simulink model "fuzzy_Control_sim"  (R2023a)
settings: Solver=VariableStepAuto  StartTime=0.0  StopTime=20  RelTol=1e-3
values from neighbouring files (symbols this model uses):
  c = 2050    [PID_Controller.m]    (also in set_Fun.m)
  ks = 60000    [PID_Controller.m]    (also in set_Fun.m)
  kt = 362000    [PID_Controller.m]    (also in set_Fun.m)
  ms = 1173    [PID_Controller.m]    (also in set_Fun.m)
  mu = 152.1    [PID_Controller.m]    (also in set_Fun.m)
undefined symbols (not defined in the file or in its folder): c0
libraries: fuzblock x2
settings Model: Creator=Administrator  LastModifiedBy=Administrator

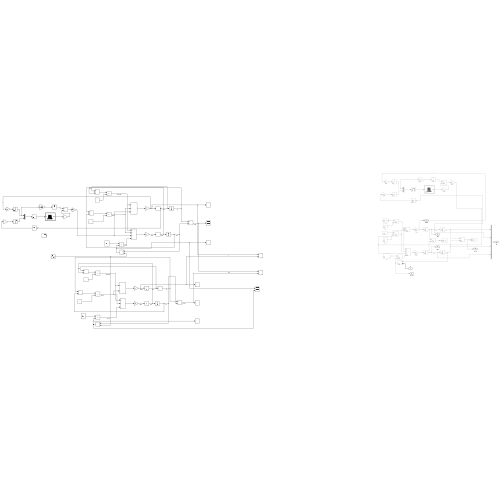
[thumbnail: Simulink's stored preview of the top-level diagram]
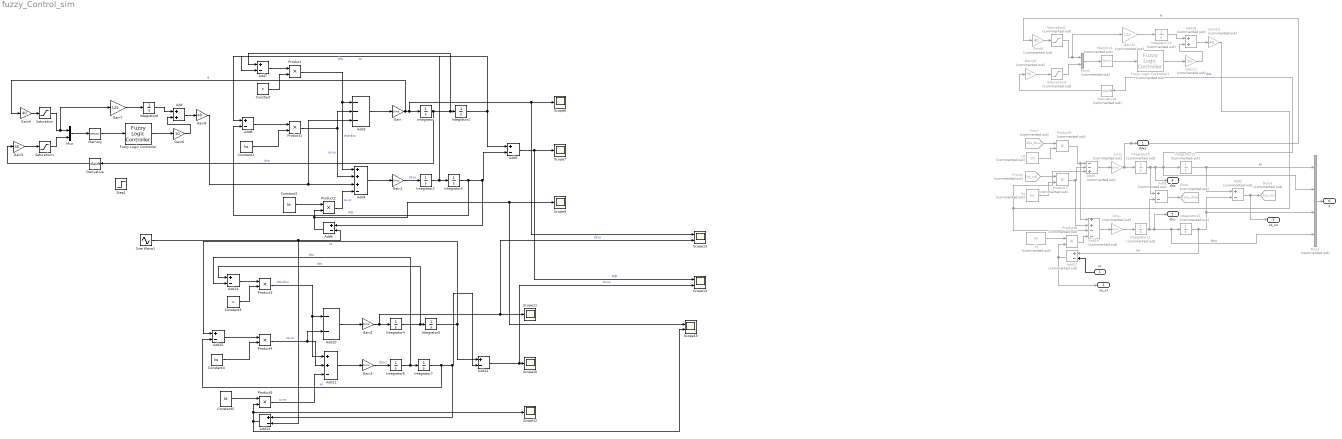
== system fuzzy_Control_sim ==
  xr : Inport
  1/ms : Gain  Commented=on  Gain=1/ms
  1/mu : Gain  Commented=on  Gain=1/mu
  Add : Sum
  Add1 : Sum  Commented=on  Inputs=+-
  Add10 : Sum  Inputs=--
  Add11 : Sum  Inputs=++-
  Add{5..8,12..15} (8 alike) : Sum  Inputs=+-
  Add16 : Sum  Commented=on  Inputs=++--
  Add17 : Sum  Commented=on  Inputs=+-
  Add18 : Sum  Commented=on
  Add2 : Sum  Commented=on  Inputs=+-
  Add3 : Sum  Inputs=---
  Add4 : Sum  Inputs=+++-
  Add9 : Sum  Commented=on  Inputs=--+
  Constant : Constant  Value=c
  Constant1 : Constant  Value=ks
  Constant2 : Constant  Value=kt
  Constant3 : Constant  Value=c
  Constant4 : Constant  Value=ks
  Constant5 : Constant  Value=kt
  Derivative : Derivative
  Derivative1 : Derivative  Commented=on
  From : From  Commented=on  GotoTag=dxs_dxu
  From2 : From  Commented=on  GotoTag=xs_xu
  Fuzzy Logic Controller : fuzblock/Fuzzy Logic  Controller  FIS='fuzzy_Model_1.fis'  OutputSampleNumber=101  DataType=double  FuzzifiedInputs=off  RuleFiringStrengths=off  RuleOutputs=off  AggregatedOutputs=off  SimulateUsing=Interpreted execution  OutOfRangeInputValueMessage=warning  NoRuleFiredMessage=warning  EmptyOutputFuzzySetMessage=warning
  Fuzzy Logic Controller1 : fuzblock/Fuzzy Logic  Controller  Commented=on  FIS='fuzzy_Model_1.fis'  OutputSampleNumber=101  DataType=double  FuzzifiedInputs=off  RuleFiringStrengths=off  RuleOutputs=off  AggregatedOutputs=off  SimulateUsing=Interpreted execution  OutOfRangeInputValueMessage=warning  NoRuleFiredMessage=warning  EmptyOutputFuzzySetMessage=warning
  Gain : Gain  Gain=1/ms
  Gain1 : Gain  Gain=1/mu
  Gain10 : Gain  Commented=on  Gain=30
  Gain11 : Gain  Commented=on  Gain=10
  Gain12 : Gain  Commented=on  Gain=125
  Gain13 : Gain  Commented=on  Gain=40
  Gain2 : Gain  Gain=1/ms
  Gain3 : Gain  Gain=1/mu
  Gain4 : Gain  Gain=40
  Gain5 : Gain  Gain=30
  Gain6 : Gain  Gain=10
  Gain7 : Gain  Gain=125
  Gain8 : Gain  Gain=40
  Gain9 : Gain  Commented=on  Gain=40
  Goto : Goto  Commented=on  GotoTag=dxs_dxu
  Goto1 : Goto  Commented=on  GotoTag=xs_xu
  Integrator{,1..8} (9 alike) : Integrator
  Integrator{9..13} (5 alike) : Integrator  Commented=on
  Memory : Memory  InitialCondition=1
  Memory1 : Memory  Commented=on  InitialCondition=1
  Mux : Mux  Inputs=2
  Mux1 : Mux  Commented=on
  Mux2 : Mux  Commented=on  Inputs=2
  Product{,1..5} (6 alike) : Product
  Product6 : Product  Commented=on
  Product7 : Product  Commented=on
  Product8 : Product  Commented=on
  Saturation : Saturate  UpperLimit=3  LowerLimit=-3
  Saturation1 : Saturate  UpperLimit=3  LowerLimit=-3
  Saturation2 : Saturate  Commented=on  UpperLimit=3  LowerLimit=-3
  Saturation3 : Saturate  Commented=on  UpperLimit=3  LowerLimit=-3
  Scope{7..12} (6 alike) : Scope
  Scope13 : Scope  NumInputPorts=2
  Scope14 : Scope  NumInputPorts=2
  Scope15 : Scope  NumInputPorts=2
  Sine Wave1 : Sin  Amplitude=0.05  Frequency=2*pi  SampleTime=0
  Step1 : Step  Time=0.1  SampleTime=0
  c0 : Constant  Commented=on  Value=c0
  ks : Constant  Commented=on  Value=ks
  kt : Constant  Commented=on  Value=kt
  ddxs : Outport
  xu_xr : Outport  Port=2
  xs_xu : Outport  Port=3
  dxs : Outport  Port=4
  dxu : Outport  Port=5
  X : Outport  Port=6
  wires:
  Add3/1 -> Gain/1
  Add4/1 -> Gain1/1
  Gain/1 -> Integrator/1, Scope13/1, Scope8/1, Gain4/1  "e"
  Gain1/1 -> Integrator2/1  "d2xu"
  Integrator2/1 -> Add7/2, Integrator3/1  "dxu"
  Integrator1/1 -> Add5/1, Add8/1  "xs"
  Integrator3/1 -> Add6/1, Add5/2, Add8/2  "PID"
  Add5/1 -> Scope14/1, Scope7/1  "PID"
  Constant/1 -> Product/2
  Constant1/1 -> Product1/2
  Constant2/1 -> Product2/1
  Add6/1 -> Scope15/1, Scope9/1, Product2/2
  Product2/1 -> Add4/4  "xu-xr"
  Product/1 -> Add4/1, Add3/1  "dxs-dxu"
  Product1/1 -> Add4/2, Add3/2  "xs-xu"
  Add7/1 -> Product/1
  Add8/1 -> Product1/1
  Sine Wave1/1 -> Add6/2, Add13/2
  Integrator4/1 -> Add14/1, Integrator5/1  "dxs"
  Add10/1 -> Gain2/1
  Integrator6/1 -> Add14/2, Integrator7/1  "dxu"
  Product4/1 -> Add11/2, Add10/2  "xs-xu"
  Gain2/1 -> Scope13/2, Scope11/1, Integrator4/1  "d2xs"
  Constant5/1 -> Product5/1
  Gain3/1 -> Integrator6/1  "d2xu"
  Integrator7/1 -> Add15/2, Add13/1, Add12/2  "xu"
  Add14/1 -> Product3/1
  Add11/1 -> Gain3/1
  Product5/1 -> Add11/3  "xu-xr"
  Constant4/1 -> Product4/2
  Constant3/1 -> Product3/2
  Product3/1 -> Add11/1, Add10/1  "dxs-dxu"
  Add15/1 -> Product4/1
  Add12/1 -> Scope14/2, Scope10/1  "xs-xu"
  Integrator5/1 -> Add12/1, Add15/1  "xs"
  Memory/1 -> Fuzzy Logic Controller/1
  Mux/1 -> Memory/1
  Fuzzy Logic Controller/1 -> Gain6/1
  Derivative/1 -> Gain5/1
  Gain4/1 -> Saturation/1
  Gain5/1 -> Saturation1/1
  Add/1 -> Gain8/1
  Saturation1/1 -> Mux/2
  Gain7/1 -> Integrator8/1
  Saturation/1 -> Gain7/1, Mux/1
  Integrator8/1 -> Add/1
  Gain6/1 -> Add/2
  Gain8/1 -> Add4/3, Add3/3
  Add13/1 -> Product5/2, Scope12/1, Scope15/2
  Mux1/1 -> X/1
  Add17/1 -> xu_xr/1, Product8/2
  Product8/1 -> Add16/4
  Add2/1 -> xs_xu/1, Goto1/1
  Add1/1 -> Goto/1
  From2/1 -> Product7/1
  Product6/1 -> Add16/1, Add9/1
  ks/1 -> Product7/2
  Integrator11/1 -> Add1/2, dxu/1, Mux1/4, Integrator12/1  "dxu"
  Product7/1 -> Add16/2, Add9/2
  xr/1 -> Add17/2
  From/1 -> Product6/1
  c0/1 -> Product6/2
  Add16/1 -> 1/mu/1
  Add9/1 -> 1/ms/1
  Integrator12/1 -> Add17/1, Mux1/3, Add2/2  "xu"
  Integrator9/1 -> Mux1/2, Derivative1/1, Integrator10/1, dxs/1, Add1/1  "dxs"
  Integrator10/1 -> Mux1/1, Add2/1  "xs"
  1/mu/1 -> Integrator11/1
  kt/1 -> Product8/1
  Integrator/1 -> Add7/1, Integrator1/1, Derivative/1  "dxs"
  1/ms/1 -> Gain9/1, ddxs/1, Integrator9/1  "e"
  Gain12/1 -> Integrator13/1
  Saturation2/1 -> Gain12/1, Mux2/1
  Gain11/1 -> Add18/2
  Gain13/1 -> Add9/3, Add16/3
  Saturation3/1 -> Mux2/2
  Add18/1 -> Gain13/1
  Derivative1/1 -> Gain10/1
  Gain9/1 -> Saturation2/1
  Gain10/1 -> Saturation3/1
  Mux2/1 -> Memory1/1
  Fuzzy Logic Controller1/1 -> Gain11/1
  Memory1/1 -> Fuzzy Logic Controller1/1
  Integrator13/1 -> Add18/1
